simulink model "Stinger"  (R2020a)
settings: Solver=ode15s  StartTime=0.0  StopTime=10  RelTol=1e-3  EnableMultiTasking=on
undefined symbols (not defined in the file): a, Fuselage, J, Ke, kt, kv, LeftAftArm, LeftAftBall, LeftAftProp, LeftAftSkid, LeftArm, LeftArms, LeftFrontArm, LeftFrontBall, LeftFrontProp, LeftFrontSkid, LeftProp, LeftSkids, R, RightAftArm, RightAftBall, RightAftProp, RightAftSkid, RightArm, RightArms, RightFrontArm, RightFrontBall, RightFrontProp, RightFrontSkid, RightProp, RightSkids, sigbuilder_block, w0, X, Y, Z
libraries: sm_lib x167, nesl_utility x70
(part 3 of 4)

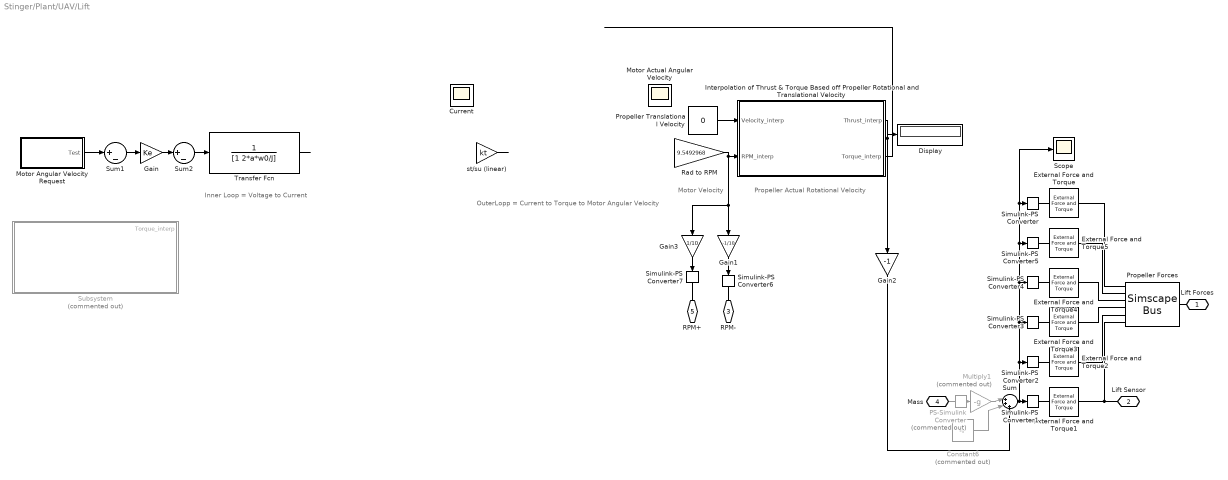
== system Stinger/Plant/UAV/Lift ==
  note: Inner Loop = Voltage to Current
  note: OuterLopp = Current to Torque to Motor Angular Velocity
  note: Motor Velocity
  note: Propeller Actual Rotational Velocity
  Constant6 : Constant  Commented=on  Value=-F
  Current : Scope
  Display : Display
  External Force and Torque{,1..5} (6 alike) : sm_lib/Forces and Torques/External Force and Torque  ForceResolutionFrame=AttachedFrame  EnableForceX=on  EnableForceY=off  EnableForceZ=off  EnableForce=off  TorqueResolutionFrame=AttachedFrame  EnableTorqueX=off  EnableTorqueY=off  EnableTorqueZ=off  EnableTorque=off
  Gain : Gain  Gain=Ke
  Gain1 : Gain  Gain=-1/10
  Gain2 : Gain  Gain=-1
  Gain3 : Gain  Gain=1/10
  Interpolation of Thrust & Torque Based off Propeller Rotational and Translational Velocity : MATLAB Function  TreatAsAtomicUnit=on
  Motor Actual Angular Velocity : Scope
  Motor Angular Velocity Request : Subsystem  Tag=STV Subsys  LoadFcn=sigbuilder_block('load');  StartFcn=sigbuilder_block('start');  StopFcn=sigbuilder_block('stop');  ClipboardFcn=sigbuilder_block('clipboard');  mask(Sigbuilder block){tuvar=[0:10]}
      mask help: Simulink:masks:SigbuilderBlock_MD
      mask init:
      | if ~strcmp(get_param(bdroot(gcbh),'SimulationStatus'),'stopped') tuvar = sigbuilder_block('maskInit'); end
      settings: CopyFcn=sigbuilder_block('copy');  DeleteFcn=sigbuilder_block('delete');  ModelCloseFcn=sigbuilder_block('modelClose');  PreSaveFcn=sigbuilder_block('preSave');  PauseFcn=sigbuilder_block('pause');  ContinueFcn=sigbuilder_block('continue');  NameChangeFcn=sigbuilder_block('namechange');  OpenFcn=sigbuilder_block('open',[144 129.75 551.25 399.75 ]);  CloseFcn=sigbuilder_block('close');
      mask Display: plot(0, 0, 100, 100,[2, 2, 32, 32, 2], [68, 8, 8, 68, 68],[32, 2], [38, 38], [32, 19, 2],[53, 60, 44], [32, 17, 17, 2],[16, 16, 31, 31]);txt = getActiveGroup(gcbh);text(2, 100, txt,'verticalAlignment', 'top');
  Multiply1 : Gain  Commented=on  Gain=-g
  PS-Simulink Converter : nesl_utility/PS-Simulink Converter  Commented=on  PhysicalDomain=network_engine_domain  SubClassName=ps_output  LeftPortType=input  RightPortType=output  PseudoPeriodic=off  Frequencies=[]  Unit=inherit  AffineConversion=off
  Propeller Forces : SimscapeBus  HierarchyStrings=LeftAftProp;LeftProp;LeftFrontProp;RightFrontProp;RightProp;RightAftProp
  Propeller Translational Velocity : Constant  Value=0  SampleTime=-1
  Rad to RPM : Gain  Gain=9.5492968
  Scope : Scope
  Simulink-PS Converter{,1..5} (6 alike) : nesl_utility/Simulink-PS Converter  PhysicalDomain=network_engine_domain  SubClassName=ps_input  LeftPortType=input  RightPortType=output  PseudoPeriodic=off  Frequencies=[]  NoiseDistribution=none  NoiseParameters=[]  Unit=N  AffineConversion=off  FilteringAndDerivatives=provide  SimscapeFilterOrder=1  InputFilterTimeConstant=0.001  UdotUserProvided=0
  Simulink-PS Converter6 : nesl_utility/Simulink-PS Converter  PhysicalDomain=network_engine_domain  SubClassName=ps_input  LeftPortType=input  RightPortType=output  PseudoPeriodic=off  Frequencies=[]  NoiseDistribution=none  NoiseParameters=[]  Unit=1  AffineConversion=off  FilteringAndDerivatives=filter  SimscapeFilterOrder=2  InputFilterTimeConstant=0.001  UdotUserProvided=0
  Simulink-PS Converter7 : nesl_utility/Simulink-PS Converter  PhysicalDomain=network_engine_domain  SubClassName=ps_input  LeftPortType=input  RightPortType=output  PseudoPeriodic=off  Frequencies=[]  NoiseDistribution=none  NoiseParameters=[]  Unit=1  AffineConversion=off  FilteringAndDerivatives=filter  SimscapeFilterOrder=2  InputFilterTimeConstant=0.001  UdotUserProvided=0
  Subsystem : Subsystem  Commented=on
  Sum : Sum  Inputs=|+++
  Sum1 : Sum  Inputs=|+-
  Sum2 : Sum  Inputs=|+-
  Transfer Fcn : TransferFcn  Denominator=[1 2*a*w0/J]
  st/su (linear) : Gain  Gain=kt
  Lift Forces : PMIOPort  Side=Left
  Lift Sensor : PMIOPort  Port=2  Side=Left
  RPM- : PMIOPort  Port=3  Side=Right
  Mass : PMIOPort  Port=4  Side=Right
  RPM+ : PMIOPort  Port=5  Side=Right
  wires:
  PS-Simulink Converter/1 -> Multiply1/1
  Multiply1/1 -> Sum/1
  Interpolation of Thrust & Torque Based off Propeller Rotational and Translational Velocity/1(Thrust_interp) -> Gain2/1, Display/1
  Motor Angular Velocity Request/1(Test) -> Sum1/1
  Rad to RPM/1 -> Gain3/1, Gain1/1, Interpolation of Thrust & Torque Based off Propeller Rotational and Translational Velocity/2(RPM_interp)
  Sum2/1 -> Transfer Fcn/1
  Transfer Fcn/1 -> ?
  Propeller Translational Velocity/1 -> Interpolation of Thrust & Torque Based off Propeller Rotational and Translational Velocity/1(Velocity_interp)
  Sum1/1 -> Gain/1
  ? -> Sum2/2, st/su (linear)/1, Current/1
  ? -> Rad to RPM/1, Motor Actual Angular Velocity/1, Sum1/2
  st/su (linear)/1 -> ?
  Gain/1 -> Sum2/1
  Constant6/1 -> Sum/2
  Sum/1 -> Simulink-PS Converter2/1, Simulink-PS Converter3/1, Simulink-PS Converter4/1, Simulink-PS Converter5/1, Scope/1, Simulink-PS Converter/1, Simulink-PS Converter1/1
  Gain1/1 -> Simulink-PS Converter6/1
  Gain2/1 -> Sum/3
  Gain3/1 -> Simulink-PS Converter7/1
  Interpolation of Thrust & Torque Based off Propeller Rotational and Translational Velocity/2(Torque_interp) -> ?
  connections:
  Propeller Forces/RConn1 -- Lift Forces/RConn1
  Simulink-PS Converter1/RConn1 -- External Force and Torque1/LConn1
  Simulink-PS Converter2/RConn1 -- External Force and Torque2/LConn1
  Simulink-PS Converter4/RConn1 -- External Force and Torque4/LConn1
  Simulink-PS Converter3/RConn1 -- External Force and Torque3/LConn1
  Simulink-PS Converter5/RConn1 -- External Force and Torque5/LConn1
  External Force and Torque/LConn1 -- Simulink-PS Converter/RConn1
  Propeller Forces/LConn1 -- External Force and Torque/RConn1
  PS-Simulink Converter/LConn1 -- Mass/RConn1
  Propeller Forces/LConn6 -- Lift Sensor/RConn1 -- External Force and Torque1/RConn1
  External Force and Torque2/RConn1 -- Propeller Forces/LConn5
  Propeller Forces/LConn4 -- External Force and Torque3/RConn1
  Propeller Forces/LConn3 -- External Force and Torque4/RConn1
  Propeller Forces/LConn2 -- External Force and Torque5/RConn1
  Simulink-PS Converter6/RConn1 -- RPM-/RConn1
  Simulink-PS Converter7/RConn1 -- RPM+/RConn1

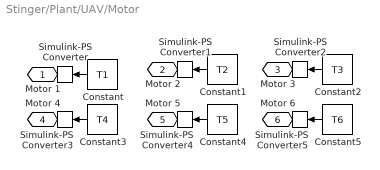
== system Stinger/Plant/UAV/Motor ==
  Constant : Constant  Value=T1
  Constant1 : Constant  Value=T2
  Constant2 : Constant  Value=T3
  Constant3 : Constant  Value=T4
  Constant4 : Constant  Value=T5
  Constant5 : Constant  Value=T6
  Simulink-PS Converter{,1..5} (6 alike) : nesl_utility/Simulink-PS Converter  PhysicalDomain=network_engine_domain  SubClassName=ps_input  LeftPortType=input  RightPortType=output  PseudoPeriodic=off  Frequencies=[]  NoiseDistribution=none  NoiseParameters=[]  Unit=1  AffineConversion=off  FilteringAndDerivatives=provide  SimscapeFilterOrder=1  InputFilterTimeConstant=0.001  UdotUserProvided=0
  Motor 1 : PMIOPort  Side=Right
  Motor 2 : PMIOPort  Port=2  Side=Right
  Motor 3 : PMIOPort  Port=3  Side=Right
  Motor 4 : PMIOPort  Port=4  Side=Right
  Motor 5 : PMIOPort  Port=5  Side=Right
  Motor 6 : PMIOPort  Port=6  Side=Right
  wires:
  Constant/1 -> Simulink-PS Converter/1
  Constant5/1 -> Simulink-PS Converter5/1
  Constant4/1 -> Simulink-PS Converter4/1
  Constant3/1 -> Simulink-PS Converter3/1
  Constant2/1 -> Simulink-PS Converter2/1
  Constant1/1 -> Simulink-PS Converter1/1
  connections:
  Motor 1/RConn1 -- Simulink-PS Converter/RConn1
  Motor 6/RConn1 -- Simulink-PS Converter5/RConn1
  Simulink-PS Converter3/RConn1 -- Motor 4/RConn1
  Motor 3/RConn1 -- Simulink-PS Converter2/RConn1
  Motor 2/RConn1 -- Simulink-PS Converter1/RConn1
  Motor 5/RConn1 -- Simulink-PS Converter4/RConn1

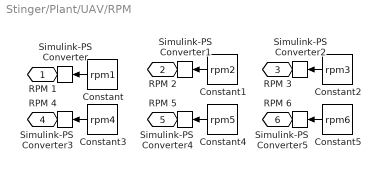
== system Stinger/Plant/UAV/RPM ==
  Constant : Constant  Value=rpm1
  Constant1 : Constant  Value=rpm2
  Constant2 : Constant  Value=rpm3
  Constant3 : Constant  Value=rpm4
  Constant4 : Constant  Value=rpm5
  Constant5 : Constant  Value=rpm6
  Simulink-PS Converter{,1..5} (6 alike) : nesl_utility/Simulink-PS Converter  PhysicalDomain=network_engine_domain  SubClassName=ps_input  LeftPortType=input  RightPortType=output  PseudoPeriodic=off  Frequencies=[]  NoiseDistribution=none  NoiseParameters=[]  Unit=1  AffineConversion=off  FilteringAndDerivatives=provide  SimscapeFilterOrder=1  InputFilterTimeConstant=0.001  UdotUserProvided=0
  RPM 1 : PMIOPort  Side=Right
  RPM 2 : PMIOPort  Port=2  Side=Right
  RPM 3 : PMIOPort  Port=3  Side=Right
  RPM 4 : PMIOPort  Port=4  Side=Right
  RPM 5 : PMIOPort  Port=5  Side=Right
  RPM 6 : PMIOPort  Port=6  Side=Right
  wires:
  Constant1/1 -> Simulink-PS Converter1/1
  Constant2/1 -> Simulink-PS Converter2/1
  Constant3/1 -> Simulink-PS Converter3/1
  Constant4/1 -> Simulink-PS Converter4/1
  Constant5/1 -> Simulink-PS Converter5/1
  Constant/1 -> Simulink-PS Converter/1
  connections:
  RPM 5/RConn1 -- Simulink-PS Converter4/RConn1
  RPM 2/RConn1 -- Simulink-PS Converter1/RConn1
  RPM 3/RConn1 -- Simulink-PS Converter2/RConn1
  Simulink-PS Converter3/RConn1 -- RPM 4/RConn1
  RPM 6/RConn1 -- Simulink-PS Converter5/RConn1
  RPM 1/RConn1 -- Simulink-PS Converter/RConn1

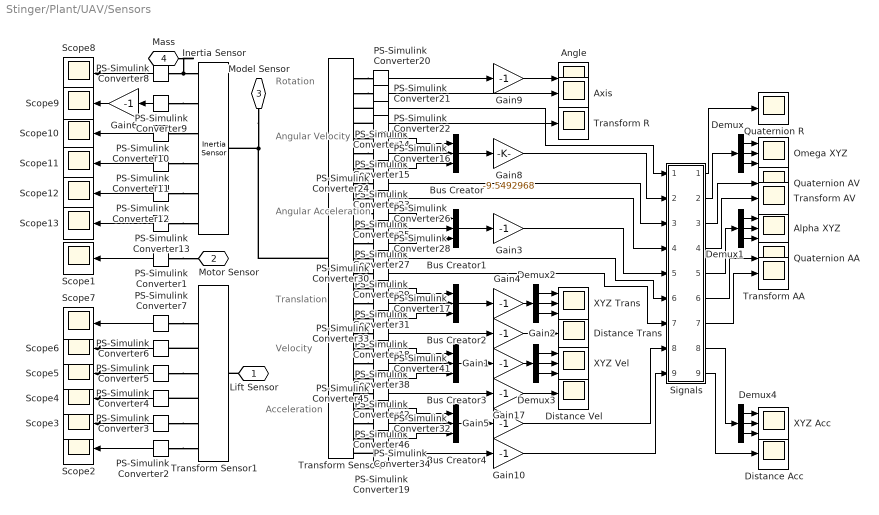
== system Stinger/Plant/UAV/Sensors ==
  note: Rotation
  note: Angular Velocity
  note: Angular Acceleration
  note: Translation
  note: Velocity
  note: Acceleration
  Alpha XYZ : Scope  NumInputPorts=3
  Angle : Scope
  Axis : Scope
  Bus Creator{,1..4} (5 alike) : BusCreator  Inputs=3
  Demux{,1..4} (5 alike) : Demux  Outputs=3
  Distance Acc : Scope
  Distance Trans : Scope
  Distance Vel : Scope
  Gain{1..6,9..10,17} (9 alike) : Gain  Gain=-1
  Gain8 : Gain  Gain=-9.5492968
  Inertia Sensor : sm_lib/Body Elements/Inertia Sensor  SensorExtent=BodyGroup  SpanWeldJoints=off  ExcludeGroundedBodies=off  MeasurementFrame=Attached  SenseMass=on  SenseCenterOfMass=on  SenseInertiaMatrix=on  SenseCenteredInertiaMatrix=on  SensePrincipalInertiaMatrix=on  SenseRotationMatrix=on  GraphicType=None  PrincipalInertiaFrameSize=20  GraphicVisPropType=SimpleVisualProperties  GraphicDiffuseColor=[0.5 0.5 0.5]  GraphicSpecularColor=[0.5 0.5 0.5 1.0]  GraphicAmbientColor=[0.15 0.15 0.15 1.0]  GraphicEmissiveColor=[0.0 0.0 0.0 1.0]  GraphicShininess=75  GraphicOpacity=1.0
      settings: SourceProductBaseCode=MS
  Omega XYZ : Scope  NumInputPorts=3
  PS-Simulink Converter{1..34,38,41..42,45..46} (39 alike) : nesl_utility/PS-Simulink Converter  PhysicalDomain=network_engine_domain  SubClassName=ps_output  LeftPortType=input  RightPortType=output  PseudoPeriodic=off  Frequencies=[]  Unit=inherit  AffineConversion=off
  Quaternion AA : Scope
  Quaternion AV : Scope
  Quaternion R : Scope
  Scope{1..13} (13 alike) : Scope
  Signals : Subsystem  mask{P=0.0075}
      mask prompts: P "Period"
  Transform Sensor1 : sm_lib/Frames and Transforms/Transform Sensor  MeasurementFrame=World  SenseAngle=off  SenseAxis=off  SenseAngle1=off  SenseAngle2=off  SenseAngle3=off  SenseQ=off  SenseR=off  SenseOmegaX=on  SenseOmegaY=on  SenseOmegaZ=on  SenseOmega1=off  SenseOmega2=off  SenseOmega3=off  SenseQDot=off  SenseRDot=off  SenseAlphaX=off  SenseAlphaY=off  SenseAlphaZ=off  SenseAlpha1=off  SenseAlpha2=off  SenseAlpha3=off  SenseQDDot=off  SenseRDDot=off  SenseX=on  SenseY=on  SenseZ=on  SenseRad=off  SenseAzim=off  SenseDist=off  SenseInc=off  SenseXDot=off  SenseYDot=off  SenseZDot=off  SenseRadDot=off  SenseAzimDot=off  SenseDistDot=off  SenseIncDot=off  SenseXDDot=off  SenseYDDot=off  SenseZDDot=off  SenseRadDDot=off  SenseAzimDDot=off  SenseDistDDot=off  SenseIncDDot=off
  Transform Sensor2 : sm_lib/Frames and Transforms/Transform Sensor  MeasurementFrame=World  SenseAngle=on  SenseAxis=on  SenseAngle1=off  SenseAngle2=off  SenseAngle3=off  SenseQ=on  SenseR=on  SenseOmegaX=on  SenseOmegaY=on  SenseOmegaZ=on  SenseOmega1=off  SenseOmega2=off  SenseOmega3=off  SenseQDot=on  SenseRDot=on  SenseAlphaX=on  SenseAlphaY=on  SenseAlphaZ=on  SenseAlpha1=off  SenseAlpha2=off  SenseAlpha3=off  SenseQDDot=on  SenseRDDot=on  SenseX=on  SenseY=on  SenseZ=on  SenseRad=off  SenseAzim=off  SenseDist=on  SenseInc=off  SenseXDot=on  SenseYDot=on  SenseZDot=on  SenseRadDot=off  SenseAzimDot=off  SenseDistDot=on  SenseIncDot=off  SenseXDDot=on  SenseYDDot=on  SenseZDDot=on  SenseRadDDot=off  SenseAzimDDot=off  SenseDistDDot=on  SenseIncDDot=off
  Transform AA : Scope
  Transform AV : Scope
  Transform R : Scope
  XYZ Acc : Scope  NumInputPorts=3
  XYZ Trans : Scope  NumInputPorts=3
  XYZ Vel : Scope  NumInputPorts=3
  Lift Sensor : PMIOPort  Side=Left
  Motor Sensor : PMIOPort  Port=2  Side=Left
  Model Sensor : PMIOPort  Port=3  Side=Left
  Mass : PMIOPort  Port=4  Side=Right
  wires:
  PS-Simulink Converter1/1 -> Scope1/1
  PS-Simulink Converter4/1 -> Scope4/1
  PS-Simulink Converter6/1 -> Scope6/1
  PS-Simulink Converter3/1 -> Scope3/1
  PS-Simulink Converter2/1 -> Scope2/1
  PS-Simulink Converter5/1 -> Scope5/1
  PS-Simulink Converter7/1 -> Scope7/1
  PS-Simulink Converter8/1 -> Scope8/1
  PS-Simulink Converter10/1 -> Scope10/1
  PS-Simulink Converter11/1 -> Scope11/1
  PS-Simulink Converter12/1 -> Scope12/1
  PS-Simulink Converter13/1 -> Scope13/1
  PS-Simulink Converter9/1 -> Gain6/1
  Gain6/1 -> Scope9/1
  PS-Simulink Converter20/1 -> Gain9/1
  Gain9/1 -> Angle/1
  Demux/1 -> Omega XYZ/1
  Demux/2 -> Omega XYZ/2
  PS-Simulink Converter16/1 -> Bus Creator/2
  PS-Simulink Converter15/1 -> Bus Creator/1
  PS-Simulink Converter23/1 -> Bus Creator/3
  PS-Simulink Converter28/1 -> Bus Creator1/3
  PS-Simulink Converter27/1 -> Bus Creator1/2
  PS-Simulink Converter26/1 -> Bus Creator1/1
  Gain2/1 -> Distance Trans/1
  PS-Simulink Converter33/1 -> Gain2/1
  PS-Simulink Converter17/1 -> Bus Creator2/2
  PS-Simulink Converter18/1 -> Bus Creator2/3
  Demux2/1 -> XYZ Trans/1
  PS-Simulink Converter31/1 -> Bus Creator2/1
  PS-Simulink Converter46/1 -> Bus Creator4/1
  PS-Simulink Converter34/1 -> Bus Creator4/3
  PS-Simulink Converter32/1 -> Bus Creator4/2
  PS-Simulink Converter41/1 -> Bus Creator3/2
  PS-Simulink Converter42/1 -> Bus Creator3/3
  PS-Simulink Converter45/1 -> Gain17/1
  Gain17/1 -> Distance Vel/1
  PS-Simulink Converter38/1 -> Bus Creator3/1
  Demux/3 -> Omega XYZ/3
  Demux2/3 -> XYZ Trans/3
  Bus Creator/1 -> Gain8/1
  Bus Creator1/1 -> Gain3/1
  Demux1/1 -> Alpha XYZ/1
  Demux1/2 -> Alpha XYZ/2
  Demux1/3 -> Alpha XYZ/3
  Bus Creator2/1 -> Gain4/1
  PS-Simulink Converter19/1 -> Gain10/1
  PS-Simulink Converter21/1 -> Axis/1
  Demux4/1 -> XYZ Acc/1
  Demux4/2 -> XYZ Acc/2
  Demux4/3 -> XYZ Acc/3
  PS-Simulink Converter22/1 -> Transform R/1
  Bus Creator3/1 -> Gain1/1
  Bus Creator4/1 -> Gain5/1
  Gain4/1 -> Demux2/1
  Demux2/2 -> XYZ Trans/2
  Demux3/1 -> XYZ Vel/1
  Demux3/2 -> XYZ Vel/2
  Demux3/3 -> XYZ Vel/3
  Gain1/1 -> Demux3/1
  PS-Simulink Converter14/1 -> Signals/1(In1)
  Gain8/1 -> Signals/2(In2)
  PS-Simulink Converter24/1 -> Signals/3(In3)
  PS-Simulink Converter25/1 -> Signals/4(In4)
  Gain3/1 -> Signals/5(In10)
  PS-Simulink Converter29/1 -> Signals/6(In5)
  PS-Simulink Converter30/1 -> Signals/7(In6)
  Gain5/1 -> Signals/8(In7)
  Gain10/1 -> Signals/9(In8)
  Signals/1(Out1) -> Quaternion R/1
  Signals/2(Out2) -> Demux/1
  Signals/3(Out3) -> Quaternion AV/1
  Signals/4(Out4) -> Transform AV/1
  Signals/5(Out10) -> Demux1/1
  Signals/6(Out5) -> Quaternion AA/1
  Signals/7(Out6) -> Transform AA/1
  Signals/8(Out7) -> Demux4/1
  Signals/9(Out8) -> Distance Acc/1
  connections:
  PS-Simulink Converter1/LConn1 -- Motor Sensor/RConn1
  PS-Simulink Converter8/LConn1 -- Mass/RConn1 -- Inertia Sensor/RConn1
  PS-Simulink Converter9/LConn1 -- Inertia Sensor/RConn2
  PS-Simulink Converter10/LConn1 -- Inertia Sensor/RConn3
  PS-Simulink Converter11/LConn1 -- Inertia Sensor/RConn4
  PS-Simulink Converter12/LConn1 -- Inertia Sensor/RConn5
  PS-Simulink Converter13/LConn1 -- Inertia Sensor/RConn6
  PS-Simulink Converter2/LConn1 -- Transform Sensor1/RConn7
  PS-Simulink Converter3/LConn1 -- Transform Sensor1/RConn6
  Transform Sensor1/RConn5 -- PS-Simulink Converter4/LConn1
  PS-Simulink Converter5/LConn1 -- Transform Sensor1/RConn4
  Transform Sensor1/RConn3 -- PS-Simulink Converter6/LConn1
  PS-Simulink Converter7/LConn1 -- Transform Sensor1/RConn2
  Transform Sensor2/RConn2 -- PS-Simulink Converter20/LConn1
  Transform Sensor2/RConn3 -- PS-Simulink Converter21/LConn1
  PS-Simulink Converter14/LConn1 -- Transform Sensor2/RConn4
  PS-Simulink Converter22/LConn1 -- Transform Sensor2/RConn5
  Transform Sensor2/RConn6 -- PS-Simulink Converter15/LConn1
  Transform Sensor2/RConn7 -- PS-Simulink Converter16/LConn1
  Transform Sensor2/RConn8 -- PS-Simulink Converter23/LConn1
  Transform Sensor2/RConn9 -- PS-Simulink Converter24/LConn1
  Transform Sensor2/RConn10 -- PS-Simulink Converter25/LConn1
  Transform Sensor2/RConn11 -- PS-Simulink Converter26/LConn1
  Transform Sensor2/RConn12 -- PS-Simulink Converter27/LConn1
  Transform Sensor2/RConn13 -- PS-Simulink Converter28/LConn1
  Transform Sensor2/RConn14 -- PS-Simulink Converter29/LConn1
  Transform Sensor2/RConn15 -- PS-Simulink Converter30/LConn1
  Transform Sensor2/RConn16 -- PS-Simulink Converter31/LConn1
  Transform Sensor2/RConn17 -- PS-Simulink Converter17/LConn1
  Transform Sensor2/RConn18 -- PS-Simulink Converter18/LConn1
  Transform Sensor2/RConn19 -- PS-Simulink Converter33/LConn1
  Transform Sensor2/RConn20 -- PS-Simulink Converter38/LConn1
  Transform Sensor2/RConn21 -- PS-Simulink Converter41/LConn1
  Transform Sensor2/RConn22 -- PS-Simulink Converter42/LConn1
  Transform Sensor2/RConn23 -- PS-Simulink Converter45/LConn1
  Transform Sensor2/RConn24 -- PS-Simulink Converter46/LConn1
  Transform Sensor2/RConn25 -- PS-Simulink Converter32/LConn1
  Transform Sensor2/RConn26 -- PS-Simulink Converter34/LConn1
  PS-Simulink Converter19/LConn1 -- Transform Sensor2/RConn27
  Lift Sensor/RConn1 -- Transform Sensor1/LConn1
  Model Sensor/RConn1 -- Transform Sensor2/LConn1 -- Inertia Sensor/LConn1

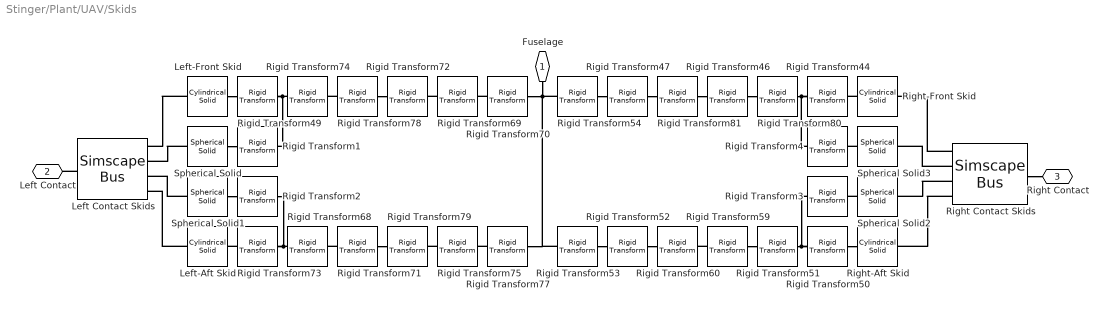
== system Stinger/Plant/UAV/Skids ==
  Left Contact Skids : SimscapeBus  HierarchyStrings=LeftFrontSkid;LeftFrontBall;LeftAftBall;LeftAftSkid
  Left-Aft Skid : sm_lib/Body Elements/Cylindrical Solid  GraphicAmbientColor=[0.15 0.15 0.15 1.0]  BasedOnType=Density  CenterOfMass=[0 0 0]  CenterOfMassUnits=m  GraphicDiffuseColor=rgb2  CylinderLength=L2  CylinderLengthUnits=m  CylinderRadius=R2  CylinderRadiusUnits=m  Density=rho2  DensityUnits=kg/m^3  DoExposeReferenceFrame=on  GraphicEmissiveColor=[0.0 0.0 0.0 1.0]  ExportEntireGeometry=on  SerializedFrames=<Frames/>  MarkerShape=Sphere  MarkerSize=10  GraphicType=FromGeometry  InertiaType=CalculateFromGeometry  Mass=1  MassUnits=kg  MomentsOfInertia=[1 1 1]  MomentsOfInertiaUnits=kg*m^2  GraphicOpacity=op2  ProductsOfInertia=[0 0 0]  ProductsOfInertiaUnits=kg*m^2  GraphicShininess=75  GraphicSpecularColor=[0.5 0.5 0.5 1.0]  GraphicVisPropType=SimpleVisualProperties
  Left-Front Skid : sm_lib/Body Elements/Cylindrical Solid  GraphicAmbientColor=[0.15 0.15 0.15 1.0]  BasedOnType=Density  CenterOfMass=[0 0 0]  CenterOfMassUnits=m  GraphicDiffuseColor=rgb2  CylinderLength=L2  CylinderLengthUnits=m  CylinderRadius=R2  CylinderRadiusUnits=m  Density=rho2  DensityUnits=kg/m^3  DoExposeReferenceFrame=on  GraphicEmissiveColor=[0.0 0.0 0.0 1.0]  ExportEntireGeometry=on  SerializedFrames=<Frames/>  MarkerShape=Sphere  MarkerSize=10  GraphicType=FromGeometry  InertiaType=CalculateFromGeometry  Mass=1  MassUnits=kg  MomentsOfInertia=[1 1 1]  MomentsOfInertiaUnits=kg*m^2  GraphicOpacity=op2  ProductsOfInertia=[0 0 0]  ProductsOfInertiaUnits=kg*m^2  GraphicShininess=75  GraphicSpecularColor=[0.5 0.5 0.5 1.0]  GraphicVisPropType=SimpleVisualProperties
  Right Contact Skids : SimscapeBus  HierarchyStrings=RightFrontSkid;RightFrontBall;RightAftBall;RightAftSkid
  Right-Aft Skid : sm_lib/Body Elements/Cylindrical Solid  GraphicAmbientColor=[0.15 0.15 0.15 1.0]  BasedOnType=Density  CenterOfMass=[0 0 0]  CenterOfMassUnits=m  GraphicDiffuseColor=rgb2  CylinderLength=L2  CylinderLengthUnits=m  CylinderRadius=R2  CylinderRadiusUnits=m  Density=rho2  DensityUnits=kg/m^3  DoExposeReferenceFrame=on  GraphicEmissiveColor=[0.0 0.0 0.0 1.0]  ExportEntireGeometry=on  SerializedFrames=<Frames/>  MarkerShape=Sphere  MarkerSize=10  GraphicType=FromGeometry  InertiaType=CalculateFromGeometry  Mass=1  MassUnits=kg  MomentsOfInertia=[1 1 1]  MomentsOfInertiaUnits=kg*m^2  GraphicOpacity=op2  ProductsOfInertia=[0 0 0]  ProductsOfInertiaUnits=kg*m^2  GraphicShininess=75  GraphicSpecularColor=[0.5 0.5 0.5 1.0]  GraphicVisPropType=SimpleVisualProperties
  Right-Front Skid : sm_lib/Body Elements/Cylindrical Solid  GraphicAmbientColor=[0.15 0.15 0.15 1.0]  BasedOnType=Density  CenterOfMass=[0 0 0]  CenterOfMassUnits=m  GraphicDiffuseColor=rgb2  CylinderLength=L2  CylinderLengthUnits=m  CylinderRadius=R2  CylinderRadiusUnits=m  Density=rho2  DensityUnits=kg/m^3  DoExposeReferenceFrame=on  GraphicEmissiveColor=[0.0 0.0 0.0 1.0]  ExportEntireGeometry=on  SerializedFrames=<Frames/>  MarkerShape=Sphere  MarkerSize=10  GraphicType=FromGeometry  InertiaType=CalculateFromGeometry  Mass=1  MassUnits=kg  MomentsOfInertia=[1 1 1]  MomentsOfInertiaUnits=kg*m^2  GraphicOpacity=op2  ProductsOfInertia=[0 0 0]  ProductsOfInertiaUnits=kg*m^2  GraphicShininess=75  GraphicSpecularColor=[0.5 0.5 0.5 1.0]  GraphicVisPropType=SimpleVisualProperties
  Rigid Transform1 : sm_lib/Frames and Transforms/Rigid Transform  TranslationMethod=StandardAxis  TranslationStandardOffset=L2-R2  TranslationLengthUnit=m  TranslationStandardAxis=+Z  TranslationCartesianOffset=0  TranslationROffset=0  TranslationROffsetUnits=m  TranslationZOffset=0  TranslationZOffsetUnits=m  TranslationThetaOffset=0  TranslationThetaOffsetUnits=deg  RotationMethod=None  RotationAngleUnits=deg  RotationStandardAxis=+Z  RotationAngle=0.0  RotationArbitraryAxis=[0 0 1]  FollAlignAxisA=+X  BaseAlignAxisA=+Y  FollAlignAxisB=+Y  BaseAlignAxisB=+Z  RotationSequenceAxes=FollowerAxes  RotationSequence=XYX  RotationSequenceAngles=[0 0 0]  RotationSequenceAnglesUnits=deg  RotationMatrix=[1 0 0; 0 1 0; 0 0 1]
  Rigid Transform2 : sm_lib/Frames and Transforms/Rigid Transform  TranslationMethod=StandardAxis  TranslationStandardOffset=L2-R2  TranslationLengthUnit=m  TranslationStandardAxis=+Z  TranslationCartesianOffset=0  TranslationROffset=0  TranslationROffsetUnits=m  TranslationZOffset=0  TranslationZOffsetUnits=m  TranslationThetaOffset=0  TranslationThetaOffsetUnits=deg  RotationMethod=None  RotationAngleUnits=deg  RotationStandardAxis=+Z  RotationAngle=0.0  RotationArbitraryAxis=[0 0 1]  FollAlignAxisA=+X  BaseAlignAxisA=+Y  FollAlignAxisB=+Y  BaseAlignAxisB=+Z  RotationSequenceAxes=FollowerAxes  RotationSequence=XYX  RotationSequenceAngles=[0 0 0]  RotationSequenceAnglesUnits=deg  RotationMatrix=[1 0 0; 0 1 0; 0 0 1]
  Rigid Transform3 : sm_lib/Frames and Transforms/Rigid Transform  TranslationMethod=StandardAxis  TranslationStandardOffset=L2-R2  TranslationLengthUnit=m  TranslationStandardAxis=-Z  TranslationCartesianOffset=0  TranslationROffset=0  TranslationROffsetUnits=m  TranslationZOffset=0  TranslationZOffsetUnits=m  TranslationThetaOffset=0  TranslationThetaOffsetUnits=deg  RotationMethod=None  RotationAngleUnits=deg  RotationStandardAxis=+Z  RotationAngle=0.0  RotationArbitraryAxis=[0 0 1]  FollAlignAxisA=+X  BaseAlignAxisA=+Y  FollAlignAxisB=+Y  BaseAlignAxisB=+Z  RotationSequenceAxes=FollowerAxes  RotationSequence=XYX  RotationSequenceAngles=[0 0 0]  RotationSequenceAnglesUnits=deg  RotationMatrix=[1 0 0; 0 1 0; 0 0 1]
  Rigid Transform4 : sm_lib/Frames and Transforms/Rigid Transform  TranslationMethod=StandardAxis  TranslationStandardOffset=L2-R2  TranslationLengthUnit=m  TranslationStandardAxis=-Z  TranslationCartesianOffset=0  TranslationROffset=0  TranslationROffsetUnits=m  TranslationZOffset=0  TranslationZOffsetUnits=m  TranslationThetaOffset=0  TranslationThetaOffsetUnits=deg  RotationMethod=None  RotationAngleUnits=deg  RotationStandardAxis=+Z  RotationAngle=0.0  RotationArbitraryAxis=[0 0 1]  FollAlignAxisA=+X  BaseAlignAxisA=+Y  FollAlignAxisB=+Y  BaseAlignAxisB=+Z  RotationSequenceAxes=FollowerAxes  RotationSequence=XYX  RotationSequenceAngles=[0 0 0]  RotationSequenceAnglesUnits=deg  RotationMatrix=[1 0 0; 0 1 0; 0 0 1]
  Rigid Transform44 : sm_lib/Frames and Transforms/Rigid Transform  TranslationMethod=StandardAxis  TranslationStandardOffset=L2/2-R2  TranslationLengthUnit=m  TranslationStandardAxis=-Z  TranslationCartesianOffset=0  TranslationROffset=0  TranslationROffsetUnits=m  TranslationZOffset=0  TranslationZOffsetUnits=m  TranslationThetaOffset=0  TranslationThetaOffsetUnits=deg  RotationMethod=None  RotationAngleUnits=deg  RotationStandardAxis=+Z  RotationAngle=0.0  RotationArbitraryAxis=[0 0 1]  FollAlignAxisA=+X  BaseAlignAxisA=+Y  FollAlignAxisB=+Y  BaseAlignAxisB=+Z  RotationSequenceAxes=FollowerAxes  RotationSequence=XYX  RotationSequenceAngles=[0 0 0]  RotationSequenceAnglesUnits=deg  RotationMatrix=[1 0 0; 0 1 0; 0 0 1]
  Rigid Transform46 : sm_lib/Frames and Transforms/Rigid Transform  TranslationMethod=None  TranslationStandardOffset=0  TranslationLengthUnit=m  TranslationStandardAxis=+Z  TranslationCartesianOffset=0  TranslationROffset=0  TranslationROffsetUnits=m  TranslationZOffset=0  TranslationZOffsetUnits=m  TranslationThetaOffset=0  TranslationThetaOffsetUnits=deg  RotationMethod=StandardAxis  RotationAngleUnits=deg  RotationStandardAxis=+Z  RotationAngle=270-ksi  RotationArbitraryAxis=[0 0 1]  FollAlignAxisA=+X  BaseAlignAxisA=+Y  FollAlignAxisB=+Y  BaseAlignAxisB=+Z  RotationSequenceAxes=FollowerAxes  RotationSequence=XYX  RotationSequenceAngles=[0 0 0]  RotationSequenceAnglesUnits=deg  RotationMatrix=[1 0 0; 0 1 0; 0 0 1]
  Rigid Transform47 : sm_lib/Frames and Transforms/Rigid Transform  TranslationMethod=Cartesian  TranslationStandardOffset=0  TranslationLengthUnit=m  TranslationStandardAxis=+Z  TranslationCartesianOffset=[-D/8 -D/8 -H/2]  TranslationROffset=0  TranslationROffsetUnits=m  TranslationZOffset=0  TranslationZOffsetUnits=m  TranslationThetaOffset=0  TranslationThetaOffsetUnits=deg  RotationMethod=None  RotationAngleUnits=deg  RotationStandardAxis=+Z  RotationAngle=0.0  RotationArbitraryAxis=[0 0 1]  FollAlignAxisA=+X  BaseAlignAxisA=+Y  FollAlignAxisB=+Y  BaseAlignAxisB=+Z  RotationSequenceAxes=FollowerAxes  RotationSequence=XYX  RotationSequenceAngles=[0 0 0]  RotationSequenceAnglesUnits=deg  RotationMatrix=[1 0 0; 0 1 0; 0 0 1]
  Rigid Transform49 : sm_lib/Frames and Transforms/Rigid Transform  TranslationMethod=StandardAxis  TranslationStandardOffset=L2/2-R2  TranslationLengthUnit=m  TranslationStandardAxis=+Z  TranslationCartesianOffset=0  TranslationROffset=0  TranslationROffsetUnits=m  TranslationZOffset=0  TranslationZOffsetUnits=m  TranslationThetaOffset=0  TranslationThetaOffsetUnits=deg  RotationMethod=None  RotationAngleUnits=deg  RotationStandardAxis=+Z  RotationAngle=0.0  RotationArbitraryAxis=[0 0 1]  FollAlignAxisA=+X  BaseAlignAxisA=+Y  FollAlignAxisB=+Y  BaseAlignAxisB=+Z  RotationSequenceAxes=FollowerAxes  RotationSequence=XYX  RotationSequenceAngles=[0 0 0]  RotationSequenceAnglesUnits=deg  RotationMatrix=[1 0 0; 0 1 0; 0 0 1]
  Rigid Transform50 : sm_lib/Frames and Transforms/Rigid Transform  TranslationMethod=StandardAxis  TranslationStandardOffset=L2/2-R2  TranslationLengthUnit=m  TranslationStandardAxis=-Z  TranslationCartesianOffset=0  TranslationROffset=0  TranslationROffsetUnits=m  TranslationZOffset=0  TranslationZOffsetUnits=m  TranslationThetaOffset=0  TranslationThetaOffsetUnits=deg  RotationMethod=None  RotationAngleUnits=deg  RotationStandardAxis=+Z  RotationAngle=0.0  RotationArbitraryAxis=[0 0 1]  FollAlignAxisA=+X  BaseAlignAxisA=+Y  FollAlignAxisB=+Y  BaseAlignAxisB=+Z  RotationSequenceAxes=FollowerAxes  RotationSequence=XYX  RotationSequenceAngles=[0 0 0]  RotationSequenceAnglesUnits=deg  RotationMatrix=[1 0 0; 0 1 0; 0 0 1]
  Rigid Transform51 : sm_lib/Frames and Transforms/Rigid Transform  TranslationMethod=None  TranslationStandardOffset=0  TranslationLengthUnit=m  TranslationStandardAxis=+Z  TranslationCartesianOffset=0  TranslationROffset=0  TranslationROffsetUnits=m  TranslationZOffset=0  TranslationZOffsetUnits=m  TranslationThetaOffset=0  TranslationThetaOffsetUnits=deg  RotationMethod=StandardAxis  RotationAngleUnits=deg  RotationStandardAxis=+Y  RotationAngle=90+phi  RotationArbitraryAxis=[0 0 1]  FollAlignAxisA=+X  BaseAlignAxisA=+Y  FollAlignAxisB=+Y  BaseAlignAxisB=+Z  RotationSequenceAxes=FollowerAxes  RotationSequence=XYX  RotationSequenceAngles=[0 0 0]  RotationSequenceAnglesUnits=deg  RotationMatrix=[1 0 0; 0 1 0; 0 0 1]
  Rigid Transform52 : sm_lib/Frames and Transforms/Rigid Transform  TranslationMethod=Cartesian  TranslationStandardOffset=0  TranslationLengthUnit=m  TranslationStandardAxis=+Z  TranslationCartesianOffset=[D/8 -D/8 -H/2]  TranslationROffset=0  TranslationROffsetUnits=m  TranslationZOffset=0  TranslationZOffsetUnits=m  TranslationThetaOffset=0  TranslationThetaOffsetUnits=deg  RotationMethod=None  RotationAngleUnits=deg  RotationStandardAxis=+Z  RotationAngle=0.0  RotationArbitraryAxis=[0 0 1]  FollAlignAxisA=+X  BaseAlignAxisA=+Y  FollAlignAxisB=+Y  BaseAlignAxisB=+Z  RotationSequenceAxes=FollowerAxes  RotationSequence=XYX  RotationSequenceAngles=[0 0 0]  RotationSequenceAnglesUnits=deg  RotationMatrix=[1 0 0; 0 1 0; 0 0 1]
  Rigid Transform{53..54,60,70,72,77,79,81} (8 alike) : sm_lib/Frames and Transforms/Rigid Transform  TranslationMethod=StandardAxis  TranslationStandardOffset=D/2  TranslationLengthUnit=m  TranslationStandardAxis=-Z  TranslationCartesianOffset=0  TranslationROffset=0  TranslationROffsetUnits=m  TranslationZOffset=0  TranslationZOffsetUnits=m  TranslationThetaOffset=0  TranslationThetaOffsetUnits=deg  RotationMethod=None  RotationAngleUnits=deg  RotationStandardAxis=+Z  RotationAngle=0.0  RotationArbitraryAxis=[0 0 1]  FollAlignAxisA=+X  BaseAlignAxisA=+Y  FollAlignAxisB=+Y  BaseAlignAxisB=+Z  RotationSequenceAxes=FollowerAxes  RotationSequence=XYX  RotationSequenceAngles=[0 0 0]  RotationSequenceAnglesUnits=deg  RotationMatrix=[1 0 0; 0 1 0; 0 0 1]
  Rigid Transform59 : sm_lib/Frames and Transforms/Rigid Transform  TranslationMethod=None  TranslationStandardOffset=0  TranslationLengthUnit=m  TranslationStandardAxis=+Z  TranslationCartesianOffset=0  TranslationROffset=0  TranslationROffsetUnits=m  TranslationZOffset=0  TranslationZOffsetUnits=m  TranslationThetaOffset=0  TranslationThetaOffsetUnits=deg  RotationMethod=StandardAxis  RotationAngleUnits=deg  RotationStandardAxis=+Z  RotationAngle=270+ksi  RotationArbitraryAxis=[0 0 1]  FollAlignAxisA=+X  BaseAlignAxisA=+Y  FollAlignAxisB=+Y  BaseAlignAxisB=+Z  RotationSequenceAxes=FollowerAxes  RotationSequence=XYX  RotationSequenceAngles=[0 0 0]  RotationSequenceAnglesUnits=deg  RotationMatrix=[1 0 0; 0 1 0; 0 0 1]
  Rigid Transform68 : sm_lib/Frames and Transforms/Rigid Transform  TranslationMethod=StandardAxis  TranslationStandardOffset=0  TranslationLengthUnit=m  TranslationStandardAxis=+Z  TranslationCartesianOffset=0  TranslationROffset=0  TranslationROffsetUnits=m  TranslationZOffset=0  TranslationZOffsetUnits=m  TranslationThetaOffset=0  TranslationThetaOffsetUnits=deg  RotationMethod=StandardAxis  RotationAngleUnits=deg  RotationStandardAxis=+Y  RotationAngle=90-phi  RotationArbitraryAxis=[0 0 1]  FollAlignAxisA=+X  BaseAlignAxisA=+Y  FollAlignAxisB=+Y  BaseAlignAxisB=+Z  RotationSequenceAxes=FollowerAxes  RotationSequence=XYX  RotationSequenceAngles=[0 0 0]  RotationSequenceAnglesUnits=deg  RotationMatrix=[1 0 0; 0 1 0; 0 0 1]
  Rigid Transform69 : sm_lib/Frames and Transforms/Rigid Transform  TranslationMethod=Cartesian  TranslationStandardOffset=0  TranslationLengthUnit=m  TranslationStandardAxis=+Z  TranslationCartesianOffset=[-D/8 D/8 -H/2]  TranslationROffset=0  TranslationROffsetUnits=m  TranslationZOffset=0  TranslationZOffsetUnits=m  TranslationThetaOffset=0  TranslationThetaOffsetUnits=deg  RotationMethod=None  RotationAngleUnits=deg  RotationStandardAxis=+Z  RotationAngle=0.0  RotationArbitraryAxis=[0 0 1]  FollAlignAxisA=+X  BaseAlignAxisA=+Y  FollAlignAxisB=+Y  BaseAlignAxisB=+Z  RotationSequenceAxes=FollowerAxes  RotationSequence=XYX  RotationSequenceAngles=[0 0 0]  RotationSequenceAnglesUnits=deg  RotationMatrix=[1 0 0; 0 1 0; 0 0 1]
  Rigid Transform71 : sm_lib/Frames and Transforms/Rigid Transform  TranslationMethod=None  TranslationStandardOffset=0  TranslationLengthUnit=m  TranslationStandardAxis=+Z  TranslationCartesianOffset=0  TranslationROffset=0  TranslationROffsetUnits=m  TranslationZOffset=0  TranslationZOffsetUnits=m  TranslationThetaOffset=0  TranslationThetaOffsetUnits=deg  RotationMethod=StandardAxis  RotationAngleUnits=deg  RotationStandardAxis=+Z  RotationAngle=270-ksi  RotationArbitraryAxis=[0 0 1]  FollAlignAxisA=+X  BaseAlignAxisA=+Y  FollAlignAxisB=+Y  BaseAlignAxisB=+Z  RotationSequenceAxes=FollowerAxes  RotationSequence=XYX  RotationSequenceAngles=[0 0 0]  RotationSequenceAnglesUnits=deg  RotationMatrix=[1 0 0; 0 1 0; 0 0 1]
  Rigid Transform73 : sm_lib/Frames and Transforms/Rigid Transform  TranslationMethod=StandardAxis  TranslationStandardOffset=L2/2-R2  TranslationLengthUnit=m  TranslationStandardAxis=+Z  TranslationCartesianOffset=0  TranslationROffset=0  TranslationROffsetUnits=m  TranslationZOffset=0  TranslationZOffsetUnits=m  TranslationThetaOffset=0  TranslationThetaOffsetUnits=deg  RotationMethod=None  RotationAngleUnits=deg  RotationStandardAxis=+Z  RotationAngle=0.0  RotationArbitraryAxis=[0 0 1]  FollAlignAxisA=+X  BaseAlignAxisA=+Y  FollAlignAxisB=+Y  BaseAlignAxisB=+Z  RotationSequenceAxes=FollowerAxes  RotationSequence=XYX  RotationSequenceAngles=[0 0 0]  RotationSequenceAnglesUnits=deg  RotationMatrix=[1 0 0; 0 1 0; 0 0 1]
  Rigid Transform74 : sm_lib/Frames and Transforms/Rigid Transform  TranslationMethod=StandardAxis  TranslationStandardOffset=0  TranslationLengthUnit=m  TranslationStandardAxis=+Z  TranslationCartesianOffset=0  TranslationROffset=0  TranslationROffsetUnits=m  TranslationZOffset=0  TranslationZOffsetUnits=m  TranslationThetaOffset=0  TranslationThetaOffsetUnits=deg  RotationMethod=StandardAxis  RotationAngleUnits=deg  RotationStandardAxis=+Y  RotationAngle=90-phi  RotationArbitraryAxis=[0 0 1]  FollAlignAxisA=+X  BaseAlignAxisA=+Y  FollAlignAxisB=+Y  BaseAlignAxisB=+Z  RotationSequenceAxes=FollowerAxes  RotationSequence=XYX  RotationSequenceAngles=[0 0 0]  RotationSequenceAnglesUnits=deg  RotationMatrix=[1 0 0; 0 1 0; 0 0 1]
  Rigid Transform75 : sm_lib/Frames and Transforms/Rigid Transform  TranslationMethod=Cartesian  TranslationStandardOffset=0  TranslationLengthUnit=m  TranslationStandardAxis=+Z  TranslationCartesianOffset=[D/8 D/8 -H/2]  TranslationROffset=0  TranslationROffsetUnits=m  TranslationZOffset=0  TranslationZOffsetUnits=m  TranslationThetaOffset=0  TranslationThetaOffsetUnits=deg  RotationMethod=None  RotationAngleUnits=deg  RotationStandardAxis=+Z  RotationAngle=0.0  RotationArbitraryAxis=[0 0 1]  FollAlignAxisA=+X  BaseAlignAxisA=+Y  FollAlignAxisB=+Y  BaseAlignAxisB=+Z  RotationSequenceAxes=FollowerAxes  RotationSequence=XYX  RotationSequenceAngles=[0 0 0]  RotationSequenceAnglesUnits=deg  RotationMatrix=[1 0 0; 0 1 0; 0 0 1]
  Rigid Transform78 : sm_lib/Frames and Transforms/Rigid Transform  TranslationMethod=StandardAxis  TranslationStandardOffset=0  TranslationLengthUnit=m  TranslationStandardAxis=+Z  TranslationCartesianOffset=0  TranslationROffset=0  TranslationROffsetUnits=m  TranslationZOffset=0  TranslationZOffsetUnits=m  TranslationThetaOffset=0  TranslationThetaOffsetUnits=deg  RotationMethod=StandardAxis  RotationAngleUnits=deg  RotationStandardAxis=+Z  RotationAngle=270+ksi  RotationArbitraryAxis=[0 0 1]  FollAlignAxisA=+X  BaseAlignAxisA=+Y  FollAlignAxisB=+Y  BaseAlignAxisB=+Z  RotationSequenceAxes=FollowerAxes  RotationSequence=XYX  RotationSequenceAngles=[0 0 0]  RotationSequenceAnglesUnits=deg  RotationMatrix=[1 0 0; 0 1 0; 0 0 1]
  Rigid Transform80 : sm_lib/Frames and Transforms/Rigid Transform  TranslationMethod=None  TranslationStandardOffset=0  TranslationLengthUnit=m  TranslationStandardAxis=+Z  TranslationCartesianOffset=0  TranslationROffset=0  TranslationROffsetUnits=m  TranslationZOffset=0  TranslationZOffsetUnits=m  TranslationThetaOffset=0  TranslationThetaOffsetUnits=deg  RotationMethod=StandardAxis  RotationAngleUnits=deg  RotationStandardAxis=+Y  RotationAngle=90+phi  RotationArbitraryAxis=[0 0 1]  FollAlignAxisA=+X  BaseAlignAxisA=+Y  FollAlignAxisB=+Y  BaseAlignAxisB=+Z  RotationSequenceAxes=FollowerAxes  RotationSequence=XYX  RotationSequenceAngles=[0 0 0]  RotationSequenceAnglesUnits=deg  RotationMatrix=[1 0 0; 0 1 0; 0 0 1]
  Spherical Solid{,1..3} (4 alike) : sm_lib/Body Elements/Spherical Solid  GraphicAmbientColor=[0.15 0.15 0.15 1.0]  BasedOnType=Density  CenterOfMass=[0 0 0]  CenterOfMassUnits=m  GraphicDiffuseColor=rgb2  Density=rho2  DensityUnits=kg/m^3  DoExposeReferenceFrame=on  GraphicEmissiveColor=[0.0 0.0 0.0 1.0]  ExportEntireGeometry=on  SerializedExposedGeometries=<ExposedGeometries><ExposedGeometry><RawGeometryId>entire</RawGeometryId><ExposedGeometryId>G</ExposedGeometryId></ExposedGeometry></ExposedGeometries>  SerializedFrames=<Frames/>  MarkerShape=Sphere  MarkerSize=10  GraphicType=FromGeometry  InertiaType=CalculateFromGeometry  Mass=1  MassUnits=kg  MomentsOfInertia=[1 1 1]  MomentsOfInertiaUnits=kg*m^2  GraphicOpacity=op2  ProductsOfInertia=[0 0 0]  ProductsOfInertiaUnits=kg*m^2  GraphicShininess=75  GraphicSpecularColor=[0.5 0.5 0.5 1.0]  SphereRadius=R2  SphereRadiusUnits=m  GraphicVisPropType=SimpleVisualProperties
  Fuselage : PMIOPort  Side=Left
  Left Contact : PMIOPort  Port=2  Side=Left
  Right Contact : PMIOPort  Port=3  Side=Left
  connections:
  Rigid Transform59/LConn1 -- Rigid Transform60/LConn1
  Rigid Transform68/RConn1 -- Rigid Transform2/RConn1 -- Rigid Transform73/RConn1
  Rigid Transform70/LConn1 -- Rigid Transform77/LConn1 -- Rigid Transform53/LConn1 -- Rigid Transform54/LConn1 -- Fuselage/RConn1
  Rigid Transform47/RConn1 -- Rigid Transform81/RConn1
  Rigid Transform54/RConn1 -- Rigid Transform47/LConn1
  Rigid Transform52/RConn1 -- Rigid Transform60/RConn1
  Rigid Transform75/RConn1 -- Rigid Transform79/RConn1
  Rigid Transform50/LConn1 -- Right-Aft Skid/RConn1
  Left-Front Skid/RConn1 -- Rigid Transform49/LConn1
  Rigid Transform59/RConn1 -- Rigid Transform51/LConn1
  Rigid Transform70/RConn1 -- Rigid Transform69/LConn1
  Rigid Transform71/LConn1 -- Rigid Transform79/LConn1
  Rigid Transform80/RConn1 -- Rigid Transform4/RConn1 -- Rigid Transform44/RConn1
  Rigid Transform73/LConn1 -- Left-Aft Skid/RConn1
  Rigid Transform78/RConn1 -- Rigid Transform74/LConn1
  Rigid Transform77/RConn1 -- Rigid Transform75/LConn1
  Rigid Transform81/LConn1 -- Rigid Transform46/LConn1
  Rigid Transform53/RConn1 -- Rigid Transform52/LConn1
  Rigid Transform51/RConn1 -- Rigid Transform3/RConn1 -- Rigid Transform50/RConn1
  Rigid Transform78/LConn1 -- Rigid Transform72/LConn1
  Rigid Transform69/RConn1 -- Rigid Transform72/RConn1
  Rigid Transform71/RConn1 -- Rigid Transform68/LConn1
  Rigid Transform46/RConn1 -- Rigid Transform80/LConn1
  Right-Front Skid/RConn1 -- Rigid Transform44/LConn1
  Rigid Transform74/RConn1 -- Rigid Transform49/RConn1 -- Rigid Transform1/RConn1
  Spherical Solid/RConn1 -- Rigid Transform1/LConn1
  Spherical Solid1/RConn1 -- Rigid Transform2/LConn1
  Spherical Solid2/RConn1 -- Rigid Transform3/LConn1
  Spherical Solid3/RConn1 -- Rigid Transform4/LConn1
  Left Contact Skids/RConn1 -- Left Contact/RConn1
  Left-Front Skid/LConn1 -- Left Contact Skids/LConn1
  Spherical Solid/LConn1 -- Left Contact Skids/LConn2
  Spherical Solid1/LConn1 -- Left Contact Skids/LConn3
  Left-Aft Skid/LConn1 -- Left Contact Skids/LConn4
  Right Contact Skids/RConn1 -- Right Contact/RConn1
  Right Contact Skids/LConn1 -- Right-Front Skid/LConn1
  Right Contact Skids/LConn2 -- Spherical Solid3/LConn1
  Right Contact Skids/LConn3 -- Spherical Solid2/LConn1
  Right Contact Skids/LConn4 -- Right-Aft Skid/LConn1

== system Stinger/Plant/UAV/Lift/Motor Angular Velocity Request ==
  Demux : Demux  Tag=STV Demux  Outputs=1
      settings: DisplayOption=none
  FromWs : FromWorkspace  Tag=STV FromWs  VariableName=tuvar
      SigBuilderData=|
      | common.afterFinalStr = 'Extrapolate'
      | common.sampleTime = 0
      | dataSet.timeRange = [0 10]
      | dataSet.name = 'Group 1'
      | sbobj.Groups.Name = 'Group 1'
      | sbobj.Groups.Signals.Name = 'Test'
      | sbobj.Groups.Signals.XData = [0 1 2 6 8 10]
      | sbobj.Groups.Signals.YData = [0 695 655 640 705 670]
  Test : Outport  Tag=STV Outport
  wires:
  Demux/1 -> Test/1
  FromWs/1 -> Demux/1

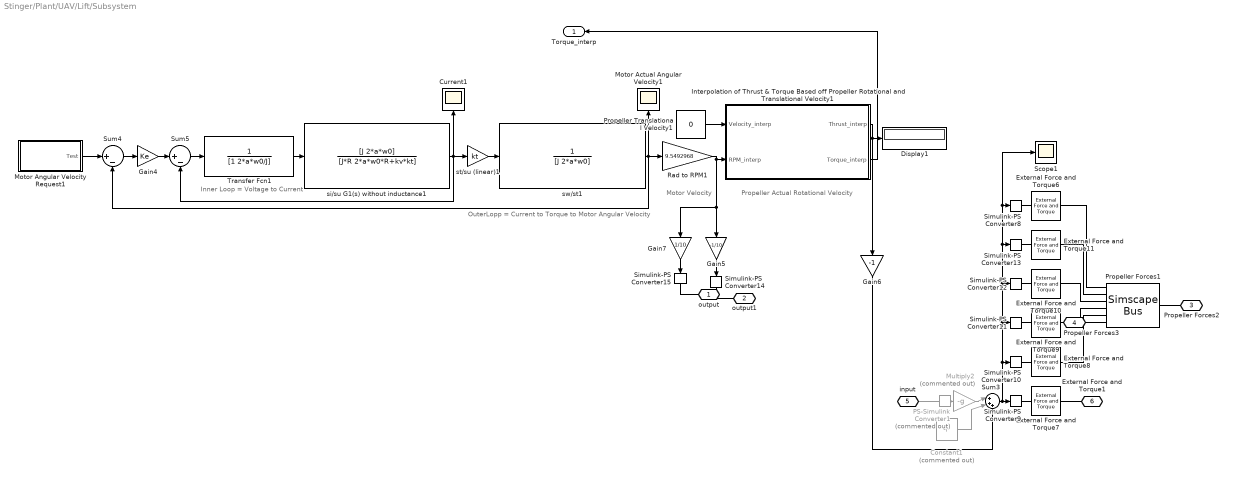
== system Stinger/Plant/UAV/Lift/Subsystem ==
  note: Inner Loop = Voltage to Current
  note: OuterLopp = Current to Torque to Motor Angular Velocity
  note: Motor Velocity
  note: Propeller Actual Rotational Velocity
  Constant1 : Constant  Commented=on  Value=-F
  Current1 : Scope
  Display1 : Display
  External Force and Torque{6..11} (6 alike) : sm_lib/Forces and Torques/External Force and Torque  ForceResolutionFrame=AttachedFrame  EnableForceX=on  EnableForceY=off  EnableForceZ=off  EnableForce=off  TorqueResolutionFrame=AttachedFrame  EnableTorqueX=off  EnableTorqueY=off  EnableTorqueZ=off  EnableTorque=off
  Gain4 : Gain  Gain=Ke
  Gain5 : Gain  Gain=-1/10
  Gain6 : Gain  Gain=-1
  Gain7 : Gain  Gain=1/10
  Interpolation of Thrust & Torque Based off Propeller Rotational and Translational Velocity1 : MATLAB Function  TreatAsAtomicUnit=on
  Motor Actual Angular Velocity1 : Scope
  Motor Angular Velocity Request1 : Subsystem  Tag=STV Subsys  LoadFcn=sigbuilder_block('load');  StartFcn=sigbuilder_block('start');  StopFcn=sigbuilder_block('stop');  ClipboardFcn=sigbuilder_block('clipboard');  mask(Sigbuilder block){tuvar=[0:10]}
      mask help: Simulink:masks:SigbuilderBlock_MD
      mask init:
      | if ~strcmp(get_param(bdroot(gcbh),'SimulationStatus'),'stopped') tuvar = sigbuilder_block('maskInit'); end
      settings: CopyFcn=sigbuilder_block('copy');  DeleteFcn=sigbuilder_block('delete');  ModelCloseFcn=sigbuilder_block('modelClose');  PreSaveFcn=sigbuilder_block('preSave');  PauseFcn=sigbuilder_block('pause');  ContinueFcn=sigbuilder_block('continue');  NameChangeFcn=sigbuilder_block('namechange');  OpenFcn=sigbuilder_block('open',[144 129.75 551.25 399.75 ]);  CloseFcn=sigbuilder_block('close');
      mask Display: plot(0, 0, 100, 100,[2, 2, 32, 32, 2], [68, 8, 8, 68, 68],[32, 2], [38, 38], [32, 19, 2],[53, 60, 44], [32, 17, 17, 2],[16, 16, 31, 31]);txt = getActiveGroup(gcbh);text(2, 100, txt,'verticalAlignment', 'top');
  Multiply2 : Gain  Commented=on  Gain=-g
  PS-Simulink Converter1 : nesl_utility/PS-Simulink Converter  Commented=on  PhysicalDomain=network_engine_domain  SubClassName=ps_output  LeftPortType=input  RightPortType=output  PseudoPeriodic=off  Frequencies=[]  Unit=inherit  AffineConversion=off
  Propeller Forces1 : SimscapeBus  HierarchyStrings=LeftAftProp;LeftProp;LeftFrontProp;RightFrontProp;RightProp;RightAftProp
  Propeller Translational Velocity1 : Constant  Value=0  SampleTime=-1
  Rad to RPM1 : Gain  Gain=9.5492968
  Scope1 : Scope
  Simulink-PS Converter{8..13} (6 alike) : nesl_utility/Simulink-PS Converter  PhysicalDomain=network_engine_domain  SubClassName=ps_input  LeftPortType=input  RightPortType=output  PseudoPeriodic=off  Frequencies=[]  NoiseDistribution=none  NoiseParameters=[]  Unit=N  AffineConversion=off  FilteringAndDerivatives=provide  SimscapeFilterOrder=1  InputFilterTimeConstant=0.001  UdotUserProvided=0
  Simulink-PS Converter14 : nesl_utility/Simulink-PS Converter  PhysicalDomain=network_engine_domain  SubClassName=ps_input  LeftPortType=input  RightPortType=output  PseudoPeriodic=off  Frequencies=[]  NoiseDistribution=none  NoiseParameters=[]  Unit=1  AffineConversion=off  FilteringAndDerivatives=filter  SimscapeFilterOrder=2  InputFilterTimeConstant=0.001  UdotUserProvided=0
  Simulink-PS Converter15 : nesl_utility/Simulink-PS Converter  PhysicalDomain=network_engine_domain  SubClassName=ps_input  LeftPortType=input  RightPortType=output  PseudoPeriodic=off  Frequencies=[]  NoiseDistribution=none  NoiseParameters=[]  Unit=1  AffineConversion=off  FilteringAndDerivatives=filter  SimscapeFilterOrder=2  InputFilterTimeConstant=0.001  UdotUserProvided=0
  Sum3 : Sum  Inputs=|+++
  Sum4 : Sum  Inputs=|+-
  Sum5 : Sum  Inputs=|+-
  Transfer Fcn1 : TransferFcn  Denominator=[1 2*a*w0/J]
  si/su G1(s) without inductance1 : TransferFcn  Numerator=[J 2*a*w0]  Denominator=[J*R 2*a*w0*R+kv*kt]
  st/su (linear)1 : Gain  Gain=kt
  sw/st1 : TransferFcn  Denominator=[J 2*a*w0]
  output : PMIOPort  Side=Right
  output1 : PMIOPort  Port=2  Side=Right
  Propeller Forces2 : PMIOPort  Port=3  Side=Right
  Propeller Forces3 : PMIOPort  Port=4  Side=Left
  input : PMIOPort  Port=5  Side=Left
  External Force and Torque1 : PMIOPort  Port=6  Side=Right
  Torque_interp : Outport
  wires:
  Interpolation of Thrust & Torque Based off Propeller Rotational and Translational Velocity1/1(Thrust_interp) -> Gain6/1, Display1/1
  st/su (linear)1/1 -> sw/st1/1
  Interpolation of Thrust & Torque Based off Propeller Rotational and Translational Velocity1/2(Torque_interp) -> Torque_interp/1
  Sum4/1 -> Gain4/1
  sw/st1/1 -> Sum4/2, Motor Actual Angular Velocity1/1, Rad to RPM1/1
  Rad to RPM1/1 -> Interpolation of Thrust & Torque Based off Propeller Rotational and Translational Velocity1/2(RPM_interp), Gain5/1, Gain7/1
  Sum3/1 -> Simulink-PS Converter9/1, Simulink-PS Converter8/1, Scope1/1, Simulink-PS Converter13/1, Simulink-PS Converter12/1, Simulink-PS Converter11/1, Simulink-PS Converter10/1
  Gain5/1 -> Simulink-PS Converter14/1
  Sum5/1 -> Transfer Fcn1/1
  Gain6/1 -> Sum3/3
  Gain7/1 -> Simulink-PS Converter15/1
  Gain4/1 -> Sum5/1
  si/su G1(s) without inductance1/1 -> Current1/1, st/su (linear)1/1, Sum5/2
  Constant1/1 -> Sum3/2
  Transfer Fcn1/1 -> si/su G1(s) without inductance1/1
  Motor Angular Velocity Request1/1(Test) -> Sum4/1
  Propeller Translational Velocity1/1 -> Interpolation of Thrust & Torque Based off Propeller Rotational and Translational Velocity1/1(Velocity_interp)
  Multiply2/1 -> Sum3/1
  PS-Simulink Converter1/1 -> Multiply2/1
  connections:
  PS-Simulink Converter1/LConn1 -- input/RConn1
  External Force and Torque8/RConn1 -- Propeller Forces1/LConn5
  Propeller Forces1/LConn2 -- External Force and Torque11/RConn1
  Propeller Forces1/LConn3 -- External Force and Torque10/RConn1
  External Force and Torque6/LConn1 -- Simulink-PS Converter8/RConn1
  Simulink-PS Converter10/RConn1 -- External Force and Torque8/LConn1
  Simulink-PS Converter9/RConn1 -- External Force and Torque7/LConn1
  Simulink-PS Converter14/RConn1 -- output1/RConn1
  Propeller Forces1/LConn4 -- External Force and Torque9/RConn1
  Simulink-PS Converter13/RConn1 -- External Force and Torque11/LConn1
  Simulink-PS Converter12/RConn1 -- External Force and Torque10/LConn1
  Simulink-PS Converter11/RConn1 -- External Force and Torque9/LConn1
  Propeller Forces1/LConn1 -- External Force and Torque6/RConn1
  Simulink-PS Converter15/RConn1 -- output/RConn1
  External Force and Torque7/RConn1 -- External Force and Torque1/RConn1
  Propeller Forces1/RConn1 -- Propeller Forces2/RConn1
  Propeller Forces1/LConn6 -- Propeller Forces3/RConn1

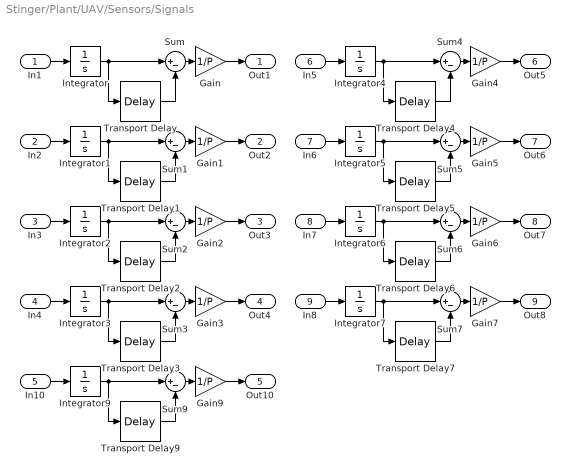
== system Stinger/Plant/UAV/Sensors/Signals ==
  In1 : Inport
  In2 : Inport  Port=2
  In3 : Inport  Port=3
  In4 : Inport  Port=4
  In10 : Inport  Port=5
  In5 : Inport  Port=6
  In6 : Inport  Port=7
  In7 : Inport  Port=8
  In8 : Inport  Port=9
  Gain{,1..7,9} (9 alike) : Gain  Gain=1/P
  Integrator{,1..7,9} (9 alike) : Integrator
  Sum{,1..7,9} (9 alike) : Sum  Inputs=|+-
  Transport Delay{,1..7,9} (9 alike) : TransportDelay  DelayTime=P  BufferSize=2048
  Out1 : Outport
  Out2 : Outport  Port=2
  Out3 : Outport  Port=3
  Out4 : Outport  Port=4
  Out10 : Outport  Port=5
  Out5 : Outport  Port=6
  Out6 : Outport  Port=7
  Out7 : Outport  Port=8
  Out8 : Outport  Port=9
  wires:
  In1/1 -> Integrator/1
  Transport Delay/1 -> Sum/2
  Integrator/1 -> Transport Delay/1, Sum/1
  Sum/1 -> Gain/1
  Gain/1 -> Out1/1
  Gain1/1 -> Out2/1
  Sum1/1 -> Gain1/1
  Integrator1/1 -> Sum1/1, Transport Delay1/1
  Transport Delay1/1 -> Sum1/2
  In2/1 -> Integrator1/1
  In3/1 -> Integrator2/1
  Transport Delay2/1 -> Sum2/2
  Integrator2/1 -> Transport Delay2/1, Sum2/1
  Sum2/1 -> Gain2/1
  Gain2/1 -> Out3/1
  Gain3/1 -> Out4/1
  Sum3/1 -> Gain3/1
  Integrator3/1 -> Sum3/1, Transport Delay3/1
  Transport Delay3/1 -> Sum3/2
  In4/1 -> Integrator3/1
  In5/1 -> Integrator4/1
  Transport Delay4/1 -> Sum4/2
  Integrator4/1 -> Transport Delay4/1, Sum4/1
  Sum4/1 -> Gain4/1
  Gain4/1 -> Out5/1
  Gain5/1 -> Out6/1
  Sum5/1 -> Gain5/1
  Integrator5/1 -> Sum5/1, Transport Delay5/1
  Transport Delay5/1 -> Sum5/2
  In6/1 -> Integrator5/1
  In7/1 -> Integrator6/1
  Transport Delay6/1 -> Sum6/2
  Integrator6/1 -> Transport Delay6/1, Sum6/1
  Sum6/1 -> Gain6/1
  Gain6/1 -> Out7/1
  Gain7/1 -> Out8/1
  Sum7/1 -> Gain7/1
  Integrator7/1 -> Sum7/1, Transport Delay7/1
  Transport Delay7/1 -> Sum7/2
  In8/1 -> Integrator7/1
  Gain9/1 -> Out10/1
  Sum9/1 -> Gain9/1
  Integrator9/1 -> Sum9/1, Transport Delay9/1
  Transport Delay9/1 -> Sum9/2
  In10/1 -> Integrator9/1

== system Stinger/Plant/UAV/Lift/Subsystem/Motor Angular Velocity Request1 ==
  Demux : Demux  Tag=STV Demux  Outputs=1
      settings: DisplayOption=none
  FromWs : FromWorkspace  Tag=STV FromWs  VariableName=tuvar
      SigBuilderData=|
      | common.afterFinalStr = 'Extrapolate'
      | common.sampleTime = 0
      | dataSet.timeRange = [0 10]
      | dataSet.name = 'Group 1'
      | sbobj.Groups.Name = 'Group 1'
      | sbobj.Groups.Signals.Name = 'Test'
      | sbobj.Groups.Signals.XData = [0 1 2 6 8 10]
      | sbobj.Groups.Signals.YData = [0 695 655 640 705 670]
  Test : Outport  Tag=STV Outport
  wires:
  FromWs/1 -> Demux/1
  Demux/1 -> Test/1
